simulink model "vjezba"  (R2017b)
settings: Solver=VariableStepAuto  StartTime=0.0  StopTime=800  RelTol=1e-3
undefined symbols (not defined in the file): ln
libraries: simulink x28
settings Model: Creator=DT User  LastModifiedBy=DT User

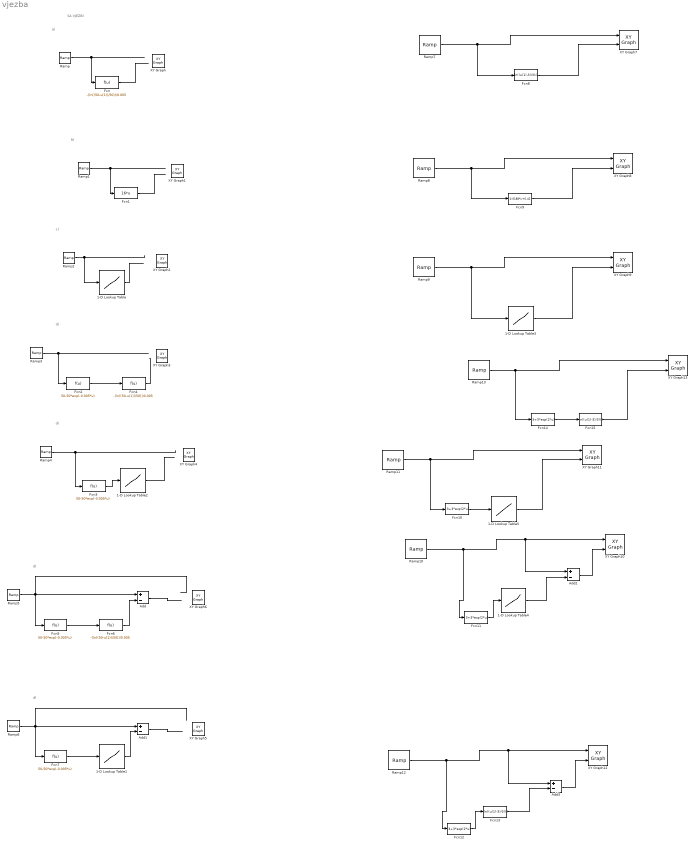
== system vjezba ==
  note: SA VJEZBI
  note: a)
  note: b)
  note: c)
  note: d)
  note: d)
  note: d)
  note: d)
  1-D Lookup Table : Lookup_n-D  NumberOfTableDimensions=1  BreakpointsForDimension1=50-50*exp(-0.005*[0:100:800])  Table=[0:100:800]  InternalRulePriority=Speed  RndMeth=Simplest  InputSameDT=on
  1-D Lookup Table1 : Lookup_n-D  NumberOfTableDimensions=1  BreakpointsForDimension1=50-50*exp(-0.005*[0:100:800])  Table=[0:100:800]  InternalRulePriority=Speed  RndMeth=Simplest  InputSameDT=on
  1-D Lookup Table2 : Lookup_n-D  NumberOfTableDimensions=1  BreakpointsForDimension1=50-50*exp(-0.005*[0:100:800])  Table=[0:100:800]  InternalRulePriority=Speed  RndMeth=Simplest  InputSameDT=on
  1-D Lookup Table3 : Lookup_n-D  NumberOfTableDimensions=1  BreakpointsForDimension1=3+3*exp(2*[0:5:50])  Table=[0:5:50]  InternalRulePriority=Speed  RndMeth=Simplest  InputSameDT=on
  1-D Lookup Table4 : Lookup_n-D  NumberOfTableDimensions=1  BreakpointsForDimension1=3+3*exp(2*[0:5:50])  Table=[0:5:50]  InternalRulePriority=Speed  RndMeth=Simplest  InputSameDT=on
  1-D Lookup Table5 : Lookup_n-D  NumberOfTableDimensions=1  BreakpointsForDimension1=3+3*exp(2*[0:5:50])  Table=[0:5:50]  InternalRulePriority=Speed  RndMeth=Simplest  InputSameDT=on
  Add{,1..3} (4 alike) : Sum  Inputs=+-
  Fcn : Fcn  Expr=-(ln((50-u(1))/50))/0.005
  Fcn1 : Fcn  Expr=16*u
  Fcn{10..12,14} (4 alike) : Fcn  Expr=3+3*exp(2*u)
  Fcn13 : Fcn  Expr=ln((u(1)-3)/3)/2
  Fcn15 : Fcn  Expr=ln((u(1)-3)/3)/2
  Fcn{2..3,5,7} (4 alike) : Fcn  Expr=50-50*exp(-0.005*u)
  Fcn4 : Fcn  Expr=-(ln((50-u(1))/50))/0.005
  Fcn6 : Fcn  Expr=-(ln((50-u(1))/50))/0.005
  Fcn8 : Fcn  Expr=ln((u(1)-3)/3)/2
  Fcn9 : Fcn  Expr=0.0188*u+0.42
  Ramp{,1..13} (14 alike) : simulink/Sources/Ramp  slope=1  start=0  X0=0
  XY Graph : simulink/Sinks/XY Graph  xmin=0  xmax=50  ymin=0  ymax=800  st=1
  XY Graph1 : simulink/Sinks/XY Graph  xmin=0  xmax=50  ymin=0  ymax=800  st=1
  XY Graph10 : simulink/Sinks/XY Graph  xmin=0  xmax=50  ymin=-10  ymax=10  st=1
  XY Graph11 : simulink/Sinks/XY Graph  xmin=0  xmax=50  ymin=-10  ymax=100  st=1
  XY Graph12 : simulink/Sinks/XY Graph  xmin=0  xmax=50  ymin=-10  ymax=10  st=1
  XY Graph13 : simulink/Sinks/XY Graph  xmin=0  xmax=50  ymin=-10  ymax=100  st=1
  XY Graph2 : simulink/Sinks/XY Graph  xmin=0  xmax=50  ymin=0  ymax=800  st=1
  XY Graph3 : simulink/Sinks/XY Graph  xmin=0  xmax=800  ymin=0  ymax=800  st=1
  XY Graph4 : simulink/Sinks/XY Graph  xmin=0  xmax=800  ymin=0  ymax=800  st=1
  XY Graph5 : simulink/Sinks/XY Graph  xmin=0  xmax=800  ymin=-10  ymax=10  st=1
  XY Graph6 : simulink/Sinks/XY Graph  xmin=0  xmax=800  ymin=-0.01  ymax=0.01  st=1
  XY Graph7 : simulink/Sinks/XY Graph  xmin=0  xmax=50  ymin=0  ymax=2  st=1
  XY Graph8 : simulink/Sinks/XY Graph  xmin=0  xmax=50  ymin=0  ymax=2  st=1
  XY Graph9 : simulink/Sinks/XY Graph  xmin=0  xmax=50  ymin=-10  ymax=10  st=1
  wires:
  Ramp/1 -> Fcn/1
  Fcn/1 -> ?
  Fcn1/1 -> ?
  Ramp1/1 -> Fcn1/1
  Ramp2/1 -> 1-D Lookup Table/1
  1-D Lookup Table/1 -> ?
  Ramp3/1 -> Fcn2/1
  Ramp4/1 -> Fcn3/1
  1-D Lookup Table2/1 -> ?
  Fcn4/1 -> ?
  Fcn2/1 -> Fcn4/1
  Fcn3/1 -> 1-D Lookup Table2/1
  Fcn5/1 -> Fcn6/1
  Ramp5/1 -> Fcn5/1, Add/1
  Fcn6/1 -> Add/2
  Add/1 -> ?
  Add1/1 -> ?
  1-D Lookup Table1/1 -> Add1/2
  Ramp6/1 -> Add1/1, Fcn7/1
  Fcn7/1 -> 1-D Lookup Table1/1
  Fcn8/1 -> XY Graph7/2
  Ramp7/1 -> Fcn8/1, XY Graph7/1
  Ramp8/1 -> XY Graph8/1, Fcn9/1
  Fcn9/1 -> XY Graph8/2
  1-D Lookup Table3/1 -> XY Graph9/2
  Ramp9/1 -> 1-D Lookup Table3/1, XY Graph9/1
  Ramp10/1 -> Fcn11/1, Add2/1, XY Graph10/1
  1-D Lookup Table4/1 -> Add2/2
  Ramp11/1 -> Fcn10/1, XY Graph11/1
  1-D Lookup Table5/1 -> XY Graph11/2
  Fcn10/1 -> 1-D Lookup Table5/1
  Add2/1 -> XY Graph10/2
  Fcn11/1 -> 1-D Lookup Table4/1
  Fcn12/1 -> Fcn13/1
  Add3/1 -> XY Graph12/2
  Fcn13/1 -> Add3/2
  Ramp12/1 -> XY Graph12/1, Add3/1, Fcn12/1
  Fcn14/1 -> Fcn15/1
  Fcn15/1 -> XY Graph13/2
  Ramp13/1 -> XY Graph13/1, Fcn14/1
